simulink model "NetworkModelNoControlTEST"  (R2018b)
settings: Solver=VariableStepAuto  StartTime=tStart  StopTime=tFinal  FixedStep=0.01  RelTol=1e-3
values from neighbouring files (symbols this model uses):
  bx = 50    [MotionModelling.m]
  by = 50    [MotionModelling.m]
  m = 1.68    [DroneSubsystemModelling.m]    (also in MotionModelling.m = 1.38)
  VelocityStarX1TEST = vx10    [MotionModelling.m]
  VelocityStarX2TEST = vx20    [MotionModelling.m]
  VelocityStarX3TEST = vx30    [MotionModelling.m]
  VelocityStarX4TEST = vx40    [MotionModelling.m]
  VelocityStarX5TEST = vx50    [MotionModelling.m]
  VelocityStarX6TEST = vx60    [MotionModelling.m]
  VelocityStarX7TEST = vx70    [MotionModelling.m]
  VelocityStarX8TEST = vx80    [MotionModelling.m]
  VelocityStarY1TEST = vy10    [MotionModelling.m]
  VelocityStarY2TEST = vy20    [MotionModelling.m]
  VelocityStarY3TEST = vy30    [MotionModelling.m]
  VelocityStarY4TEST = vy40    [MotionModelling.m]
  VelocityStarY5TEST = vy50    [MotionModelling.m]
  VelocityStarY6TEST = vy60    [MotionModelling.m]
  VelocityStarY7TEST = vy70    [MotionModelling.m]
  VelocityStarY8TEST = vy80    [MotionModelling.m]
  vx10 = vin1*cosd (theta1)    [MotionModelling.m]
  vx20 = vin2*cosd (theta2)    [MotionModelling.m]
  vx30 = vin3*cosd (theta3)    [MotionModelling.m]
  vx40 = vin4*cosd (theta4)    [MotionModelling.m]
  vx50 = vin5*cosd (theta5)    [MotionModelling.m]
  vx60 = vin6*cosd (theta6)    [MotionModelling.m]
  vx70 = vin7*cosd (theta7)    [MotionModelling.m]
  vx80 = vin2*cosd (theta8)    [MotionModelling.m]
  vy10 = vin1*sind (theta1)    [MotionModelling.m]
  vy20 = vin2*sind (theta2)    [MotionModelling.m]
  vy30 = vin3*sind (theta3)    [MotionModelling.m]
  vy40 = vin4*sind (theta4)    [MotionModelling.m]
  vy50 = vin5*sind (theta5)    [MotionModelling.m]
  vy60 = vin6*sind (theta6)    [MotionModelling.m]
  vy70 = vin7*sind (theta7)    [MotionModelling.m]
  vy80 = vin2*sind (theta8)    [MotionModelling.m]
  x10 = 10    [MotionModelling.m]
  x20 = 10    [MotionModelling.m]
  x30 = 0    [MotionModelling.m]
  x40 = -10    [MotionModelling.m]
  x50 = -10    [MotionModelling.m]
  x60 = -10    [MotionModelling.m]
  x70 = 0    [MotionModelling.m]
  x80 = 10    [MotionModelling.m]
  y10 = 0    [MotionModelling.m]
  y20 = 10    [MotionModelling.m]
  y30 = 10    [MotionModelling.m]
  y40 = 10    [MotionModelling.m]
  y50 = 0    [MotionModelling.m]
  y60 = -10    [MotionModelling.m]
  y70 = -10    [MotionModelling.m]
  y80 = -10    [MotionModelling.m]
libraries: simulink x16
settings Model: Creator=CowUser  LastModifiedBy=CowUser

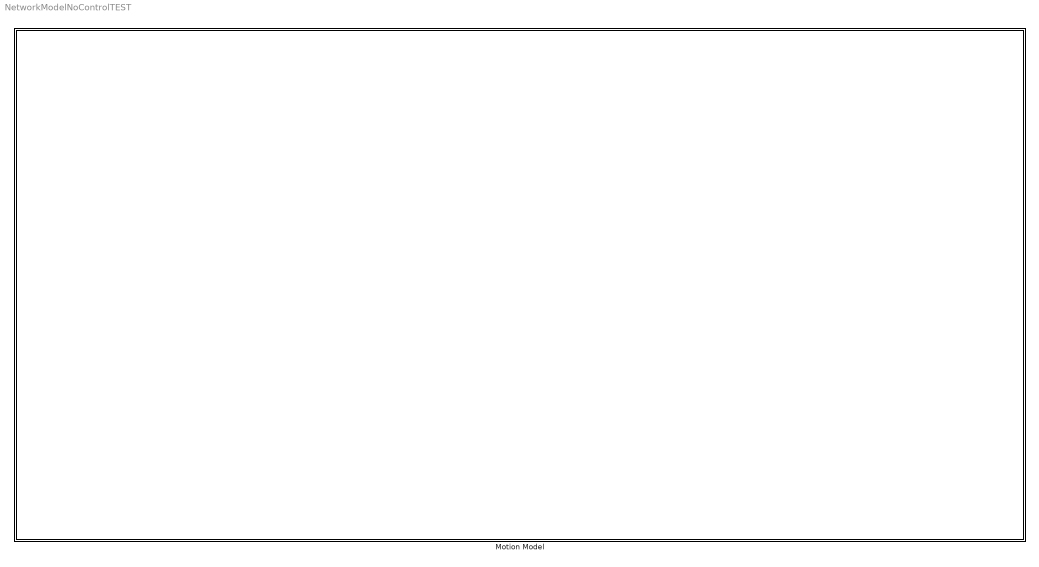
== system NetworkModelNoControlTEST ==
  Motion Model : Subsystem

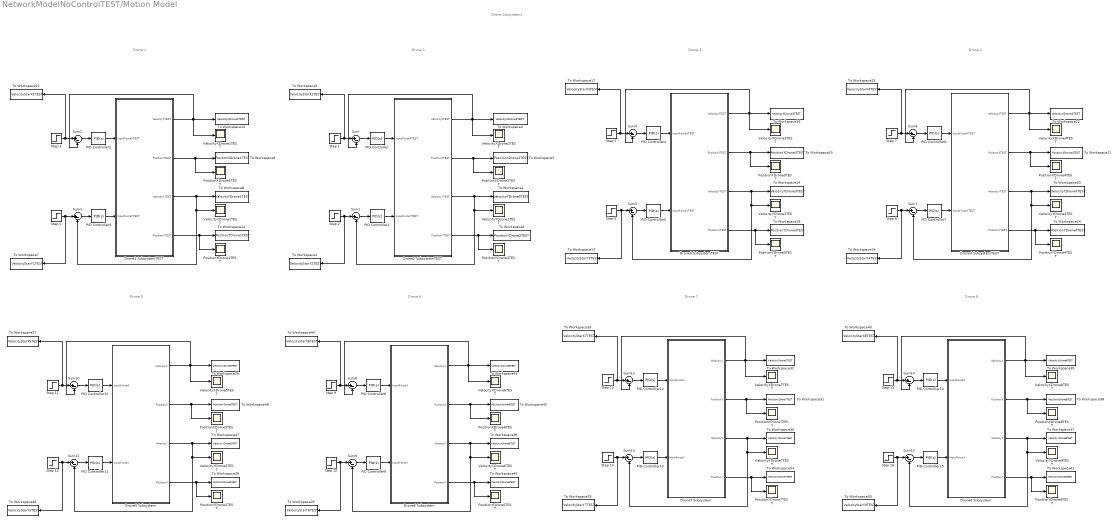
== system NetworkModelNoControlTEST/Motion Model ==
  note: Drone 1
  note: Drone 2
  note: Drone 6
  note: Drone 3
  note: Drone Subsystems
  note: Drone 4
  note: Drone 5
  note: Drone 8
  note: Drone 7
  "Drone1 SubsystemTEST " : Subsystem
  "Drone2 SubsystemTEST " : Subsystem
  "Drone3 SubsystemTEST " : Subsystem
  "Drone4 SubsystemTEST " : Subsystem
  Drone5 Subsystem : Subsystem
  Drone6 Subsystem : Subsystem
  Drone7 Subsystem : Subsystem
  Drone8 Subsystem : Subsystem
  PID Controller{,1..15} (16 alike) : simulink/Continuous/PID Controller  Controller=PID  Form=Parallel  TimeDomain=Continuous-time  SampleTime=-1  IntegratorMethod=Forward Euler  FilterMethod=Forward Euler  ControllerParametersSource=internal  P=800  I=40  D=1  UseFilter=on  N=100  TunerSelectOption=Transfer Function Based (PID Tuner App)  InitialConditionSource=internal  InitialConditionForIntegrator=0  InitialConditionForFilter=0  DifferentiatorICPrevScaledInput=0  ExternalReset=none  TrackingMode=off  Kt=1  LimitOutput=off  UpperSaturationLimit=inf  LowerSaturationLimit=-inf  LinearizeAsGain=on  AntiWindupMode=none  Kb=1  POutMin=[]  POutMax=[]  IOutMin=[]  IOutMax=[]  DOutMin=[]  DOutMax=[]  NOutMin=[]  NOutMax=[]  SumOutMin=[]  SumOutMax=[]  SaturationOutMin=[]  SaturationOutMax=[]  PParamMin=[]  PParamMax=[]  IParamMin=[]  IParamMax=[]  DParamMin=[]  DParamMax=[]  NParamMin=[]  NParamMax=[]  KbParamMin=[]  KbParamMax=[]  KtParamMin=[]  KtParamMax=[]  KbOutMin=[]  KbOutMax=[]  KtOutMin=[]  KtOutMax=[]  IntegratorOutMin=[]  IntegratorOutMax=[]  FilterOutMin=[]  FilterOutMax=[]  SumI1OutMin=[]  SumI1OutMax=[]  SumI2OutMin=[]  SumI2OutMax=[]  SumI3OutMin=[]  SumI3OutMax=[]  SumI4OutMin=[]  SumI4OutMax=[]  SumDOutMin=[]  SumDOutMax=[]  DifferentiatorOutMin=[]  DifferentiatorOutMax=[]  FilterDiffOutCoefMin=[]  FilterDiffOutCoefMax=[]  ReciprocalOutMin=[]  ReciprocalOutMax=[]  SumDenOutMin=[]  SumDenOutMax=[]  SumNumOutMin=[]  SumNumOutMax=[]  DivideOutMin=[]  DivideOutMax=[]  IntegratorContinuousStateAttributes=''  IntegratorStateMustResolveToSignalObject=off  IntegratorRTWStateStorageClass=Auto  FilterContinuousStateAttributes=''  FilterStateMustResolveToSignalObject=off  FilterRTWStateStorageClass=Auto  ParallelPVariant=InternalParameters  IdealPVariant=Disabled  IVariant=InternalParameters  DVariant=InternalParameters  IntegratorVariant=Continuous  SatVariant=Disabled  AWVariant=Passthrough  PCopyVariant=Disabled  TRVariant=Disabled  FdbkBlocksVariant=Forward  IdealPFdbkVariant=Disabled  SatFdbkVariant=Disabled  DerivativeFilterVariant=ContFilter  NVariant=InternalParameters  NCopyVariant=Disabled  FilterICVariant=InternalICsFilter  IntegratorICVariant=InternalICs  ExternalResetVariant=Disabled  TRSumVariant=Passthrough  SumFdbkVariant=Disabled  SumVariant=Sum_PID
  PositionXDrone1TEST : Scope
  PositionXDrone2TEST : Scope
  PositionXDrone3TEST : Scope
  PositionXDrone4TEST : Scope
  PositionXDrone5TEST : Scope
  PositionXDrone6TEST : Scope
  PositionXDrone7TEST : Scope
  PositionXDrone8TEST : Scope
  PositionYDrone1TEST : Scope
  PositionYDrone2TEST : Scope
  PositionYDrone3TEST : Scope
  PositionYDrone4TEST : Scope
  PositionYDrone5TEST : Scope
  PositionYDrone6TEST : Scope
  PositionYDrone7TEST : Scope
  PositionYDrone8TEST : Scope
  Step 1 : Step  Time=0  After=VelocityStarX2TEST  SampleTime=0
  Step 10 : Step  Time=0  After=VelocityStarY6TEST  SampleTime=0
  Step 11 : Step  Time=0  After=VelocityStarX5TEST  SampleTime=0
  Step 12 : Step  Time=0  After=VelocityStarY5TEST  SampleTime=0
  Step 13 : Step  Time=0  After=VelocityStarX7TEST  SampleTime=0
  Step 14 : Step  Time=0  After=VelocityStarY7TEST  SampleTime=0
  Step 15 : Step  Time=0  After=VelocityStarX8TEST  SampleTime=0
  Step 16 : Step  Time=0  After=VelocityStarY8TEST  SampleTime=0
  Step 2 : Step  Time=0  After=VelocityStarY2TEST  SampleTime=0
  Step 3 : Step  Time=0  After=VelocityStarX1TEST  SampleTime=0
  Step 4 : Step  Time=0  After=VelocityStarY1TEST  SampleTime=0
  Step 5 : Step  Time=0  After=VelocityStarX3TEST  SampleTime=0
  Step 6 : Step  Time=0  After=VelocityStarY3TEST  SampleTime=0
  Step 7 : Step  Time=0  After=VelocityStarX4TEST  SampleTime=0
  Step 8 : Step  Time=0  After=VelocityStarY4TEST  SampleTime=0
  Step 9 : Step  Time=0  After=VelocityStarX6TEST  SampleTime=0
  Sum{,1..15} (16 alike) : Sum  Inputs=|+-
  To Workspace1 : ToWorkspace  VariableName=VelocityStarY2TEST  SampleTime=-1
  To Workspace10 : ToWorkspace  VariableName=VelocityXDrone1TEST  SampleTime=-1
  To Workspace11 : ToWorkspace  VariableName=VelocityStarX1TEST  SampleTime=-1
  To Workspace12 : ToWorkspace  VariableName=PositionYDrone1TEST  SampleTime=-1
  To Workspace13 : ToWorkspace  VariableName=VelocityStarY3TEST  SampleTime=-1
  To Workspace14 : ToWorkspace  VariableName=VelocityYDrone3TEST  SampleTime=-1
  To Workspace15 : ToWorkspace  VariableName=PositionXDrone3TEST  SampleTime=-1
  To Workspace16 : ToWorkspace  VariableName=VelocityXDrone3TEST  SampleTime=-1
  To Workspace17 : ToWorkspace  VariableName=VelocityStarX3TEST  SampleTime=-1
  To Workspace18 : ToWorkspace  VariableName=PositionYDrone3TEST  SampleTime=-1
  To Workspace19 : ToWorkspace  VariableName=VelocityStarY4TEST  SampleTime=-1
  To Workspace2 : ToWorkspace  VariableName=VelocityYDrone2TEST  SampleTime=-1
  To Workspace20 : ToWorkspace  VariableName=VelocityYDrone4TEST  SampleTime=-1
  To Workspace21 : ToWorkspace  VariableName=PositionXDrone4TEST  SampleTime=-1
  To Workspace22 : ToWorkspace  VariableName=VelocityXDrone4TEST  SampleTime=-1
  To Workspace23 : ToWorkspace  VariableName=VelocityStarX4TEST  SampleTime=-1
  To Workspace24 : ToWorkspace  VariableName=PositionYDrone4TEST  SampleTime=-1
  To Workspace25 : ToWorkspace  VariableName=VelocityStarY6TEST  SampleTime=-1
  To Workspace26 : ToWorkspace  VariableName=VelocityXDrone5TEST  SampleTime=-1
  To Workspace27 : ToWorkspace  VariableName=VelocityStarX5TEST  SampleTime=-1
  To Workspace28 : ToWorkspace  VariableName=PositionYDrone5TEST  SampleTime=-1
  To Workspace29 : ToWorkspace  VariableName=VelocityStarY7TEST  SampleTime=-1
  To Workspace3 : ToWorkspace  VariableName=PositionXDrone2TEST  SampleTime=-1
  To Workspace30 : ToWorkspace  VariableName=VelocityYDrone7TEST  SampleTime=-1
  To Workspace31 : ToWorkspace  VariableName=PositionXDrone7TEST  SampleTime=-1
  To Workspace32 : ToWorkspace  VariableName=VelocityXDrone7TEST  SampleTime=-1
  To Workspace33 : ToWorkspace  VariableName=VelocityStarX7TEST  SampleTime=-1
  To Workspace34 : ToWorkspace  VariableName=PositionYDrone7TEST  SampleTime=-1
  To Workspace35 : ToWorkspace  VariableName=VelocityStarY8TEST  SampleTime=-1
  To Workspace36 : ToWorkspace  VariableName=VelocityYDrone6TEST  SampleTime=-1
  To Workspace37 : ToWorkspace  VariableName=VelocityYDrone8TEST  SampleTime=-1
  To Workspace38 : ToWorkspace  VariableName=PositionXDrone8TEST  SampleTime=-1
  To Workspace39 : ToWorkspace  VariableName=VelocityXDrone8TEST  SampleTime=-1
  To Workspace4 : ToWorkspace  VariableName=VelocityXDrone2TEST  SampleTime=-1
  To Workspace40 : ToWorkspace  VariableName=VelocityStarX8TEST  SampleTime=-1
  To Workspace41 : ToWorkspace  VariableName=PositionYDrone8TEST  SampleTime=-1
  To Workspace42 : ToWorkspace  VariableName=PositionXDrone6TEST  SampleTime=-1
  To Workspace43 : ToWorkspace  VariableName=VelocityXDrone6TEST  SampleTime=-1
  To Workspace44 : ToWorkspace  VariableName=VelocityStarX6TEST  SampleTime=-1
  To Workspace45 : ToWorkspace  VariableName=PositionYDrone6TEST  SampleTime=-1
  To Workspace46 : ToWorkspace  VariableName=VelocityStarY5TEST  SampleTime=-1
  To Workspace47 : ToWorkspace  VariableName=VelocityYDrone5TEST  SampleTime=-1
  To Workspace48 : ToWorkspace  VariableName=PositionXDrone5TEST  SampleTime=-1
  To Workspace5 : ToWorkspace  VariableName=VelocityStarX2TEST  SampleTime=-1
  To Workspace6 : ToWorkspace  VariableName=PositionYDrone2TEST  SampleTime=-1
  To Workspace7 : ToWorkspace  VariableName=VelocityStarY1TEST  SampleTime=-1
  To Workspace8 : ToWorkspace  VariableName=VelocityYDrone1TEST  SampleTime=-1
  To Workspace9 : ToWorkspace  VariableName=PositionXDrone1TEST  SampleTime=-1
  VelocityXDrone1TEST : Scope
  VelocityXDrone2TEST : Scope
  VelocityXDrone3TEST : Scope
  VelocityXDrone4TEST : Scope
  VelocityXDrone5TEST : Scope
  VelocityXDrone6TEST : Scope
  VelocityXDrone7TEST : Scope
  VelocityXDrone8TEST : Scope
  VelocityYDrone1TEST : Scope
  VelocityYDrone2TEST : Scope
  VelocityYDrone3TEST : Scope
  VelocityYDrone4TEST : Scope
  VelocityYDrone5TEST : Scope
  VelocityYDrone6TEST : Scope
  VelocityYDrone7TEST : Scope
  VelocityYDrone8TEST : Scope
  wires:
  Sum/1 -> PID Controller/1
  "Drone2 SubsystemTEST "/3(VelocityYTEST) -> Sum1/2, VelocityYDrone2TEST/1, To Workspace2/1
  Sum1/1 -> PID Controller1/1
  PID Controller/1 -> "Drone2 SubsystemTEST "/1(InputForceXTEST)
  "Drone1 SubsystemTEST "/4(PositionYTEST) -> PositionYDrone1TEST/1, To Workspace12/1
  "Drone2 SubsystemTEST "/4(PositionYTEST) -> PositionYDrone2TEST/1, To Workspace6/1
  PID Controller7/1 -> "Drone4 SubsystemTEST "/2(InputForceYTEST)
  Step 16/1 -> To Workspace35/1, Sum15/1
  Step 14/1 -> To Workspace29/1, Sum13/1
  Step 12/1 -> To Workspace46/1, Sum11/1
  "Drone2 SubsystemTEST "/2(PositionXTEST) -> PositionXDrone2TEST/1, To Workspace3/1
  Sum11/1 -> PID Controller11/1
  PID Controller6/1 -> "Drone4 SubsystemTEST "/1(InputForceXTEST)
  Drone6 Subsystem/1(VelocityX) -> Sum8/2, To Workspace43/1, VelocityXDrone6TEST/1
  Sum15/1 -> PID Controller15/1
  PID Controller8/1 -> Drone6 Subsystem/1(InputForceX)
  Step 2/1 -> To Workspace1/1, Sum1/1
  Step 9/1 -> Sum8/1, To Workspace44/1
  Step 13/1 -> Sum12/1, To Workspace33/1
  PID Controller14/1 -> Drone8 Subsystem/1(InputForceX)
  Drone6 Subsystem/3(VelocityY) -> Sum9/2, VelocityYDrone6TEST/1, To Workspace36/1
  "Drone3 SubsystemTEST "/2(PositionXTEST) -> PositionXDrone3TEST/1, To Workspace15/1
  Sum6/1 -> PID Controller6/1
  Drone6 Subsystem/2(PositionX) -> PositionXDrone6TEST/1, To Workspace42/1
  Drone8 Subsystem/2(PositionX) -> PositionXDrone8TEST/1, To Workspace38/1
  Drone7 Subsystem/3(VelocityY) -> Sum13/2, VelocityYDrone7TEST/1, To Workspace30/1
  Drone8 Subsystem/3(VelocityY) -> Sum15/2, VelocityYDrone8TEST/1, To Workspace37/1
  Sum4/1 -> PID Controller4/1
  Drone7 Subsystem/2(PositionX) -> PositionXDrone7TEST/1, To Workspace31/1
  PID Controller12/1 -> Drone7 Subsystem/1(InputForceX)
  PID Controller1/1 -> "Drone2 SubsystemTEST "/2(InputForceYTEST)
  "Drone2 SubsystemTEST "/1(VelocityXTEST) -> Sum/2, To Workspace4/1, VelocityXDrone2TEST/1
  Drone5 Subsystem/2(PositionX) -> PositionXDrone5TEST/1, To Workspace48/1
  Sum13/1 -> PID Controller13/1
  "Drone4 SubsystemTEST "/4(PositionYTEST) -> PositionYDrone4TEST/1, To Workspace24/1
  Drone7 Subsystem/4(PositionY) -> PositionYDrone7TEST/1, To Workspace34/1
  "Drone4 SubsystemTEST "/3(VelocityYTEST) -> Sum7/2, VelocityYDrone4TEST/1, To Workspace20/1
  Step 5/1 -> Sum4/1, To Workspace17/1
  "Drone4 SubsystemTEST "/1(VelocityXTEST) -> Sum6/2, To Workspace22/1, VelocityXDrone4TEST/1
  Step 7/1 -> Sum6/1, To Workspace23/1
  Sum7/1 -> PID Controller7/1
  Step 8/1 -> To Workspace19/1, Sum7/1
  PID Controller5/1 -> "Drone3 SubsystemTEST "/2(InputForceYTEST)
  PID Controller15/1 -> Drone8 Subsystem/2(InputForceY)
  "Drone3 SubsystemTEST "/4(PositionYTEST) -> PositionYDrone3TEST/1, To Workspace18/1
  "Drone1 SubsystemTEST "/1(VelocityXTEST) -> To Workspace10/1, VelocityXDrone1TEST/1, Sum2/2
  Step 4/1 -> To Workspace7/1, Sum3/1
  PID Controller3/1 -> "Drone1 SubsystemTEST "/2(InputForceYTEST)
  "Drone3 SubsystemTEST "/3(VelocityYTEST) -> Sum5/2, VelocityYDrone3TEST/1, To Workspace14/1
  Sum2/1 -> PID Controller2/1
  "Drone1 SubsystemTEST "/3(VelocityYTEST) -> Sum3/2, VelocityYDrone1TEST/1, To Workspace8/1
  Step 1/1 -> Sum/1, To Workspace5/1
  Drone5 Subsystem/4(PositionY) -> PositionYDrone5TEST/1, To Workspace28/1
  PID Controller10/1 -> Drone5 Subsystem/1(InputForceX)
  Sum9/1 -> PID Controller9/1
  Step 3/1 -> Sum2/1, To Workspace11/1
  Drone8 Subsystem/4(PositionY) -> PositionYDrone8TEST/1, To Workspace41/1
  Sum10/1 -> PID Controller10/1
  PID Controller11/1 -> Drone5 Subsystem/2(InputForceY)
  Sum3/1 -> PID Controller3/1
  Step 6/1 -> To Workspace13/1, Sum5/1
  Step 11/1 -> Sum10/1, To Workspace27/1
  Sum14/1 -> PID Controller14/1
  Step 10/1 -> To Workspace25/1, Sum9/1
  PID Controller13/1 -> Drone7 Subsystem/2(InputForceY)
  "Drone1 SubsystemTEST "/2(PositionXTEST) -> PositionXDrone1TEST/1, To Workspace9/1
  Drone5 Subsystem/3(VelocityY) -> Sum11/2, VelocityYDrone5TEST/1, To Workspace47/1
  Sum5/1 -> PID Controller5/1
  Sum12/1 -> PID Controller12/1
  PID Controller4/1 -> "Drone3 SubsystemTEST "/1(InputForceXTEST)
  "Drone4 SubsystemTEST "/2(PositionXTEST) -> PositionXDrone4TEST/1, To Workspace21/1
  PID Controller9/1 -> Drone6 Subsystem/2(InputForceY)
  Drone6 Subsystem/4(PositionY) -> PositionYDrone6TEST/1, To Workspace45/1
  Drone7 Subsystem/1(VelocityX) -> Sum12/2, To Workspace32/1, VelocityXDrone7TEST/1
  PID Controller2/1 -> "Drone1 SubsystemTEST "/1(InputForceXTEST)
  Step 15/1 -> Sum14/1, To Workspace40/1
  Drone8 Subsystem/1(VelocityX) -> Sum14/2, To Workspace39/1, VelocityXDrone8TEST/1
  Drone5 Subsystem/1(VelocityX) -> To Workspace26/1, VelocityXDrone5TEST/1, Sum10/2
  "Drone3 SubsystemTEST "/1(VelocityXTEST) -> Sum4/2, To Workspace16/1, VelocityXDrone3TEST/1
  Sum8/1 -> PID Controller8/1

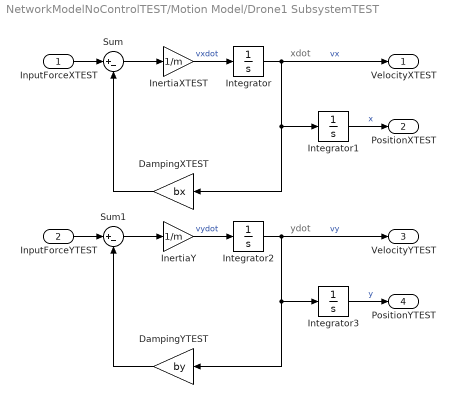
== system NetworkModelNoControlTEST/Motion Model/Drone1 SubsystemTEST  ==
  note: xdot
  note: ydot
  InputForceXTEST : Inport
  InputForceYTEST : Inport  Port=2
  "DampingXTEST " : Gain  Gain=bx
  DampingYTEST : Gain  Gain=by
  InertiaXTEST : Gain  Gain=1/m
  InertiaY : Gain  Gain=1/m
  Integrator : Integrator  InitialCondition=vx10
  Integrator1 : Integrator  InitialCondition=x10
  Integrator2 : Integrator  InitialCondition=vy10
  Integrator3 : Integrator  InitialCondition=y10
  Sum : Sum  Inputs=|+-
  Sum1 : Sum  Inputs=|+-
  VelocityXTEST : Outport
  PositionXTEST : Outport  Port=2
  VelocityYTEST : Outport  Port=3
  PositionYTEST : Outport  Port=4
  wires:
  InputForceXTEST/1 -> Sum/1
  InertiaXTEST/1 -> Integrator/1  "vxdot"
  Sum/1 -> InertiaXTEST/1
  Integrator/1 -> VelocityXTEST/1, Integrator1/1, "DampingXTEST "/1  "vx"
  "DampingXTEST "/1 -> Sum/2
  Integrator1/1 -> PositionXTEST/1  "x"
  DampingYTEST/1 -> Sum1/2
  Sum1/1 -> InertiaY/1
  InertiaY/1 -> Integrator2/1  "vydot"
  Integrator3/1 -> PositionYTEST/1  "y"
  InputForceYTEST/1 -> Sum1/1
  Integrator2/1 -> VelocityYTEST/1, Integrator3/1, DampingYTEST/1  "vy"

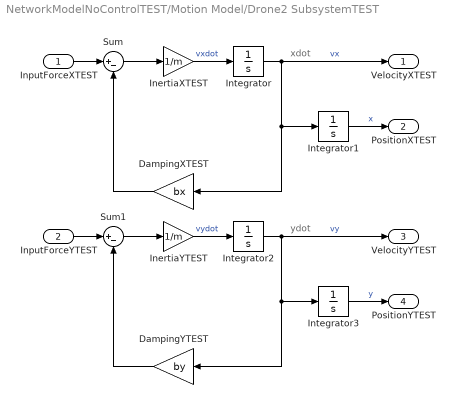
== system NetworkModelNoControlTEST/Motion Model/Drone2 SubsystemTEST  ==
  note: xdot
  note: ydot
  InputForceXTEST : Inport
  InputForceYTEST : Inport  Port=2
  "DampingXTEST " : Gain  Gain=bx
  DampingYTEST : Gain  Gain=by
  InertiaXTEST : Gain  Gain=1/m
  InertiaYTEST : Gain  Gain=1/m
  Integrator : Integrator  InitialCondition=vx20
  Integrator1 : Integrator  InitialCondition=x20
  Integrator2 : Integrator  InitialCondition=vy20
  Integrator3 : Integrator  InitialCondition=y20
  Sum : Sum  Inputs=|+-
  Sum1 : Sum  Inputs=|+-
  VelocityXTEST : Outport
  PositionXTEST : Outport  Port=2
  VelocityYTEST : Outport  Port=3
  PositionYTEST : Outport  Port=4
  wires:
  InputForceXTEST/1 -> Sum/1
  InertiaXTEST/1 -> Integrator/1  "vxdot"
  Sum/1 -> InertiaXTEST/1
  Integrator/1 -> VelocityXTEST/1, Integrator1/1, "DampingXTEST "/1  "vx"
  "DampingXTEST "/1 -> Sum/2
  Integrator1/1 -> PositionXTEST/1  "x"
  DampingYTEST/1 -> Sum1/2
  Sum1/1 -> InertiaYTEST/1
  InertiaYTEST/1 -> Integrator2/1  "vydot"
  Integrator3/1 -> PositionYTEST/1  "y"
  InputForceYTEST/1 -> Sum1/1
  Integrator2/1 -> VelocityYTEST/1, Integrator3/1, DampingYTEST/1  "vy"

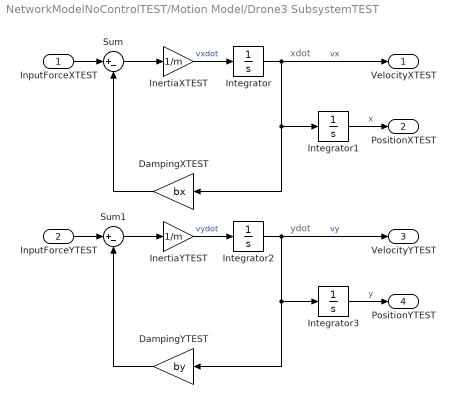
== system NetworkModelNoControlTEST/Motion Model/Drone3 SubsystemTEST  ==
  note: xdot
  note: ydot
  InputForceXTEST : Inport
  InputForceYTEST : Inport  Port=2
  "DampingXTEST " : Gain  Gain=bx
  DampingYTEST : Gain  Gain=by
  InertiaXTEST : Gain  Gain=1/m
  InertiaYTEST : Gain  Gain=1/m
  Integrator : Integrator  InitialCondition=vx30
  Integrator1 : Integrator  InitialCondition=x30
  Integrator2 : Integrator  InitialCondition=vy30
  Integrator3 : Integrator  InitialCondition=y30
  Sum : Sum  Inputs=|+-
  Sum1 : Sum  Inputs=|+-
  VelocityXTEST : Outport
  PositionXTEST : Outport  Port=2
  VelocityYTEST : Outport  Port=3
  PositionYTEST : Outport  Port=4
  wires:
  InputForceXTEST/1 -> Sum/1
  InertiaXTEST/1 -> Integrator/1  "vxdot"
  Sum/1 -> InertiaXTEST/1
  Integrator/1 -> VelocityXTEST/1, Integrator1/1, "DampingXTEST "/1  "vx"
  "DampingXTEST "/1 -> Sum/2
  Integrator1/1 -> PositionXTEST/1  "x"
  DampingYTEST/1 -> Sum1/2
  Sum1/1 -> InertiaYTEST/1
  InertiaYTEST/1 -> Integrator2/1  "vydot"
  Integrator3/1 -> PositionYTEST/1  "y"
  InputForceYTEST/1 -> Sum1/1
  Integrator2/1 -> VelocityYTEST/1, Integrator3/1, DampingYTEST/1  "vy"

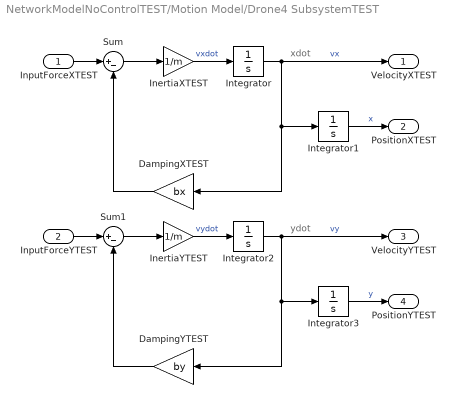
== system NetworkModelNoControlTEST/Motion Model/Drone4 SubsystemTEST  ==
  note: xdot
  note: ydot
  InputForceXTEST : Inport
  InputForceYTEST : Inport  Port=2
  "DampingXTEST " : Gain  Gain=bx
  DampingYTEST : Gain  Gain=by
  InertiaXTEST : Gain  Gain=1/m
  InertiaYTEST : Gain  Gain=1/m
  Integrator : Integrator  InitialCondition=vx40
  Integrator1 : Integrator  InitialCondition=x40
  Integrator2 : Integrator  InitialCondition=vy40
  Integrator3 : Integrator  InitialCondition=y40
  Sum : Sum  Inputs=|+-
  Sum1 : Sum  Inputs=|+-
  VelocityXTEST : Outport
  PositionXTEST : Outport  Port=2
  VelocityYTEST : Outport  Port=3
  PositionYTEST : Outport  Port=4
  wires:
  InputForceXTEST/1 -> Sum/1
  InertiaXTEST/1 -> Integrator/1  "vxdot"
  Sum/1 -> InertiaXTEST/1
  Integrator/1 -> VelocityXTEST/1, Integrator1/1, "DampingXTEST "/1  "vx"
  "DampingXTEST "/1 -> Sum/2
  Integrator1/1 -> PositionXTEST/1  "x"
  DampingYTEST/1 -> Sum1/2
  Sum1/1 -> InertiaYTEST/1
  InertiaYTEST/1 -> Integrator2/1  "vydot"
  Integrator3/1 -> PositionYTEST/1  "y"
  InputForceYTEST/1 -> Sum1/1
  Integrator2/1 -> VelocityYTEST/1, Integrator3/1, DampingYTEST/1  "vy"

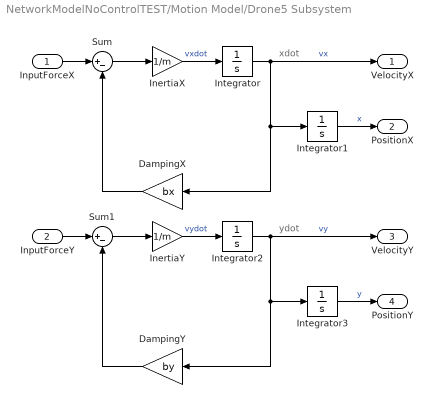
== system NetworkModelNoControlTEST/Motion Model/Drone5 Subsystem ==
  note: xdot
  note: ydot
  InputForceX : Inport
  InputForceY : Inport  Port=2
  "DampingX " : Gain  Gain=bx
  DampingY : Gain  Gain=by
  InertiaX : Gain  Gain=1/m
  InertiaY : Gain  Gain=1/m
  Integrator : Integrator  InitialCondition=vx50
  Integrator1 : Integrator  InitialCondition=x50
  Integrator2 : Integrator  InitialCondition=vy50
  Integrator3 : Integrator  InitialCondition=y50
  Sum : Sum  Inputs=|+-
  Sum1 : Sum  Inputs=|+-
  VelocityX : Outport
  PositionX : Outport  Port=2
  VelocityY : Outport  Port=3
  PositionY : Outport  Port=4
  wires:
  InputForceX/1 -> Sum/1
  InertiaX/1 -> Integrator/1  "vxdot"
  Sum/1 -> InertiaX/1
  Integrator/1 -> VelocityX/1, Integrator1/1, "DampingX "/1  "vx"
  "DampingX "/1 -> Sum/2
  Integrator1/1 -> PositionX/1  "x"
  DampingY/1 -> Sum1/2
  Sum1/1 -> InertiaY/1
  InertiaY/1 -> Integrator2/1  "vydot"
  Integrator3/1 -> PositionY/1  "y"
  InputForceY/1 -> Sum1/1
  Integrator2/1 -> VelocityY/1, Integrator3/1, DampingY/1  "vy"

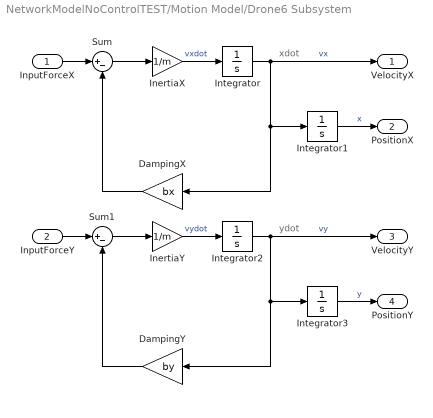
== system NetworkModelNoControlTEST/Motion Model/Drone6 Subsystem ==
  note: xdot
  note: ydot
  InputForceX : Inport
  InputForceY : Inport  Port=2
  "DampingX " : Gain  Gain=bx
  DampingY : Gain  Gain=by
  InertiaX : Gain  Gain=1/m
  InertiaY : Gain  Gain=1/m
  Integrator : Integrator  InitialCondition=vx60
  Integrator1 : Integrator  InitialCondition=x60
  Integrator2 : Integrator  InitialCondition=vy60
  Integrator3 : Integrator  InitialCondition=y60
  Sum : Sum  Inputs=|+-
  Sum1 : Sum  Inputs=|+-
  VelocityX : Outport
  PositionX : Outport  Port=2
  VelocityY : Outport  Port=3
  PositionY : Outport  Port=4
  wires:
  InputForceX/1 -> Sum/1
  InertiaX/1 -> Integrator/1  "vxdot"
  Sum/1 -> InertiaX/1
  Integrator/1 -> VelocityX/1, Integrator1/1, "DampingX "/1  "vx"
  "DampingX "/1 -> Sum/2
  Integrator1/1 -> PositionX/1  "x"
  DampingY/1 -> Sum1/2
  Sum1/1 -> InertiaY/1
  InertiaY/1 -> Integrator2/1  "vydot"
  Integrator3/1 -> PositionY/1  "y"
  InputForceY/1 -> Sum1/1
  Integrator2/1 -> VelocityY/1, Integrator3/1, DampingY/1  "vy"

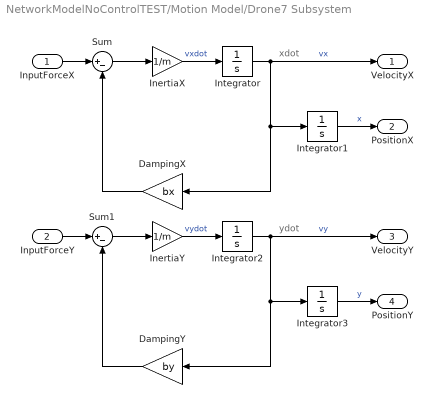
== system NetworkModelNoControlTEST/Motion Model/Drone7 Subsystem ==
  note: xdot
  note: ydot
  InputForceX : Inport
  InputForceY : Inport  Port=2
  "DampingX " : Gain  Gain=bx
  DampingY : Gain  Gain=by
  InertiaX : Gain  Gain=1/m
  InertiaY : Gain  Gain=1/m
  Integrator : Integrator  InitialCondition=vx70
  Integrator1 : Integrator  InitialCondition=x70
  Integrator2 : Integrator  InitialCondition=vy70
  Integrator3 : Integrator  InitialCondition=y70
  Sum : Sum  Inputs=|+-
  Sum1 : Sum  Inputs=|+-
  VelocityX : Outport
  PositionX : Outport  Port=2
  VelocityY : Outport  Port=3
  PositionY : Outport  Port=4
  wires:
  InputForceX/1 -> Sum/1
  InertiaX/1 -> Integrator/1  "vxdot"
  Sum/1 -> InertiaX/1
  Integrator/1 -> VelocityX/1, Integrator1/1, "DampingX "/1  "vx"
  "DampingX "/1 -> Sum/2
  Integrator1/1 -> PositionX/1  "x"
  DampingY/1 -> Sum1/2
  Sum1/1 -> InertiaY/1
  InertiaY/1 -> Integrator2/1  "vydot"
  Integrator3/1 -> PositionY/1  "y"
  InputForceY/1 -> Sum1/1
  Integrator2/1 -> VelocityY/1, Integrator3/1, DampingY/1  "vy"

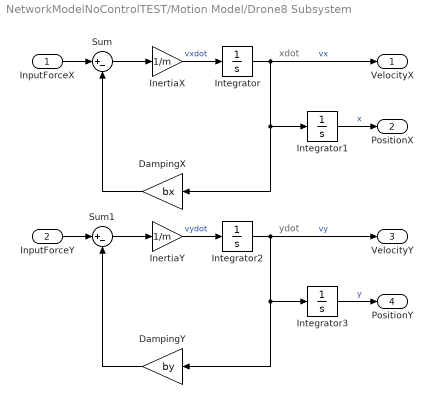
== system NetworkModelNoControlTEST/Motion Model/Drone8 Subsystem ==
  note: xdot
  note: ydot
  InputForceX : Inport
  InputForceY : Inport  Port=2
  "DampingX " : Gain  Gain=bx
  DampingY : Gain  Gain=by
  InertiaX : Gain  Gain=1/m
  InertiaY : Gain  Gain=1/m
  Integrator : Integrator  InitialCondition=vx80
  Integrator1 : Integrator  InitialCondition=x80
  Integrator2 : Integrator  InitialCondition=vy80
  Integrator3 : Integrator  InitialCondition=y80
  Sum : Sum  Inputs=|+-
  Sum1 : Sum  Inputs=|+-
  VelocityX : Outport
  PositionX : Outport  Port=2
  VelocityY : Outport  Port=3
  PositionY : Outport  Port=4
  wires:
  InputForceX/1 -> Sum/1
  InertiaX/1 -> Integrator/1  "vxdot"
  Sum/1 -> InertiaX/1
  Integrator/1 -> VelocityX/1, Integrator1/1, "DampingX "/1  "vx"
  "DampingX "/1 -> Sum/2
  Integrator1/1 -> PositionX/1  "x"
  DampingY/1 -> Sum1/2
  Sum1/1 -> InertiaY/1
  InertiaY/1 -> Integrator2/1  "vydot"
  Integrator3/1 -> PositionY/1  "y"
  InputForceY/1 -> Sum1/1
  Integrator2/1 -> VelocityY/1, Integrator3/1, DampingY/1  "vy"
